simulink model "stepFn2"  (R2024a)
settings: Solver=VariableStepAuto  StartTime=0.0  StopTime=10.0  RelTol=1e-3
settings Model: Creator=pouya  LastModifiedBy=pouya

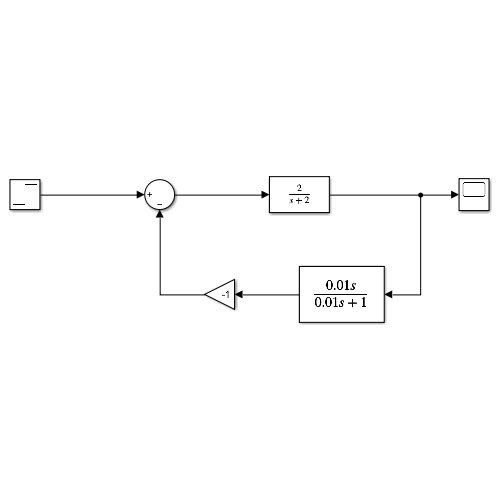
[thumbnail: Simulink's stored preview of the top-level diagram]
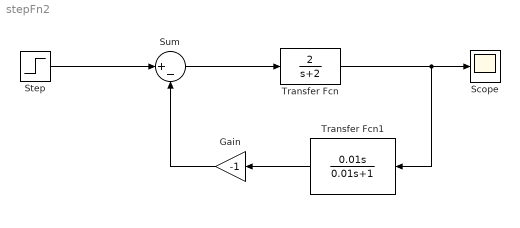
== system stepFn2 ==
  Gain : Gain  Gain=-1
  Scope : Scope
  Step : Step  Time=0  SampleTime=0
  Sum : Sum  Inputs=|+-
  Transfer Fcn : TransferFcn  Numerator=[2]  Denominator=[1 2]
  Transfer Fcn1 : TransferFcn  Numerator=[0.01 0]  Denominator=[0.01 1]  ParameterTunability=Unconstrained
  wires:
  Transfer Fcn/1 -> Transfer Fcn1/1, Scope/1
  Step/1 -> Sum/1
  Sum/1 -> Transfer Fcn/1
  Gain/1 -> Sum/2
  Transfer Fcn1/1 -> Gain/1
